simulink model "rrc_filters"  (R2013a)
settings: Solver=ode45  StartTime=0.0  StopTime=14  RelTol=1e-3
PreLoadFcn:
  | Num
libraries: dspsrcs4 x5, dsparch4 x5, dspsigops x5
settings Model: Creator=lcrockett  LastModifiedBy=hebin
settings DataIOCC: SignalLoggingSaveFormat=ModelDataLogs
settings OptimizationCC: ExpressionDepthLimit=2147483647  InitFltsAndDblsToZero=on
settings DebuggingCC: SaveWithParameterizedLinksMsg=none  FcnCallInpInsideContextMsg=UseLocalSettings  StrictBusMsg=Warning
settings GRTTargetCC: TargetFcnLib=ansi_tfl_tmw.mat  CombineOutputUpdateFcns=off  GRTInterface=on

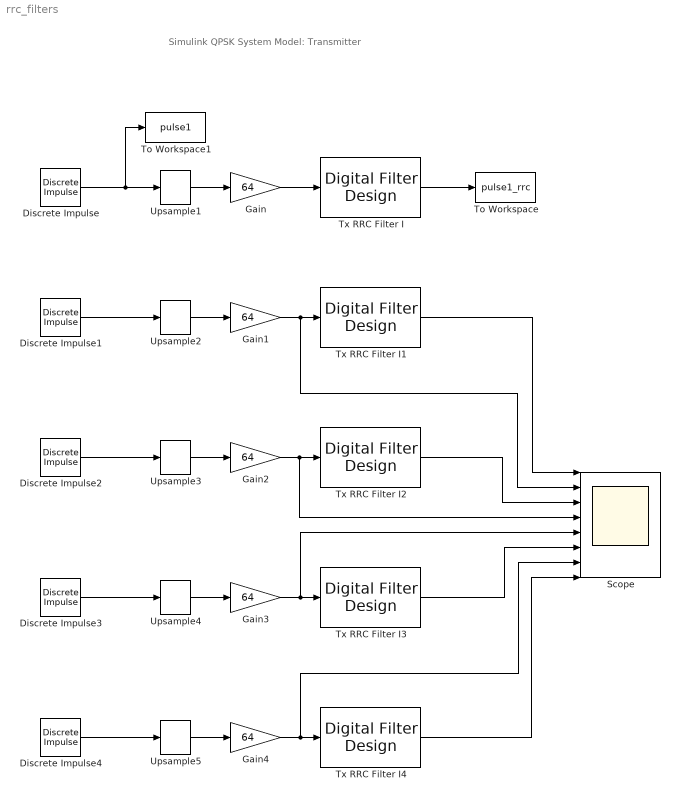
== system rrc_filters ==
  note: Simulink QPSK System Model: Transmitter
  Discrete Impulse : dspsrcs4/Discrete  Impulse  Delay=1  SampleTime=1  FrameSample=1  dataType=double  isSigned=on  wordLen=16  udDataType=sfix(16)  fracBitsMode=Best precision  numFracBits=15  OutDataTypeStr=double  LastOutDataTypeStr=double
  Discrete Impulse1 : dspsrcs4/Discrete  Impulse  Delay=2  SampleTime=1  FrameSample=1  dataType=double  isSigned=on  wordLen=16  udDataType=sfix(16)  fracBitsMode=Best precision  numFracBits=15  OutDataTypeStr=double  LastOutDataTypeStr=double
  Discrete Impulse2 : dspsrcs4/Discrete  Impulse  Delay=3  SampleTime=1  FrameSample=1  dataType=double  isSigned=on  wordLen=16  udDataType=sfix(16)  fracBitsMode=Best precision  numFracBits=15  OutDataTypeStr=double  LastOutDataTypeStr=double
  Discrete Impulse3 : dspsrcs4/Discrete  Impulse  Delay=4  SampleTime=1  FrameSample=1  dataType=double  isSigned=on  wordLen=16  udDataType=sfix(16)  fracBitsMode=Best precision  numFracBits=15  OutDataTypeStr=double  LastOutDataTypeStr=double
  Discrete Impulse4 : dspsrcs4/Discrete  Impulse  Delay=5  SampleTime=1  FrameSample=1  dataType=double  isSigned=on  wordLen=16  udDataType=sfix(16)  fracBitsMode=Best precision  numFracBits=15  OutDataTypeStr=double  LastOutDataTypeStr=double
  Gain{,1..4} (5 alike) : Gain  Gain=64
  Scope : Scope  NumInputPorts=8
      settings: YMin=-5~-5~-5~-5~-5~-5~-5~-5  YMax=5~5~5~5~5~5~5~5
  To Workspace : ToWorkspace  VariableName=pulse1_rrc  SampleTime=-1
  To Workspace1 : ToWorkspace  VariableName=pulse1  SampleTime=-1
  Tx RRC Filter I{,1..4} (5 alike) : dsparch4/Digital Filter Design  mwdsp_browser_bugfix_var=off
  Upsample{1..5} (5 alike) : dspsigops/Upsample  N=64  phase=0  InputProcessing=Inherited (this choice will be removed - see release notes)  RateOptions=Allow multirate processing  ic=0  mode=Unused parameter value
  wires:
  Tx RRC Filter I/1 -> To Workspace/1
  Discrete Impulse/1 -> Upsample1/1, To Workspace1/1
  Upsample1/1 -> Gain/1
  Gain/1 -> Tx RRC Filter I/1
  Discrete Impulse1/1 -> Upsample2/1
  Upsample2/1 -> Gain1/1
  Gain1/1 -> Scope/2, Tx RRC Filter I1/1
  Discrete Impulse2/1 -> Upsample3/1
  Upsample3/1 -> Gain2/1
  Gain2/1 -> Scope/4, Tx RRC Filter I2/1
  Discrete Impulse3/1 -> Upsample4/1
  Upsample4/1 -> Gain3/1
  Gain3/1 -> Scope/5, Tx RRC Filter I3/1
  Discrete Impulse4/1 -> Upsample5/1
  Upsample5/1 -> Gain4/1
  Gain4/1 -> Scope/7, Tx RRC Filter I4/1
  Tx RRC Filter I1/1 -> Scope/1
  Tx RRC Filter I2/1 -> Scope/3
  Tx RRC Filter I3/1 -> Scope/6
  Tx RRC Filter I4/1 -> Scope/8
